simulink model "BlockDprob2f"  (R2016b)
settings: Solver=VariableStepAuto  StartTime=0.0  StopTime=230.0  RelTol=1e-3
values from neighbouring files (symbols this model uses):
  A = [-0.322, 0.052, 0.028, -1.12 , 0.002;       0     , 0    , 1    , -0.001,     0;       -10.6 , 0    , -2.87, 0.46  , -0.65;       6.87  , 0    , -0.04, -0.32 , -0.02;       0     , 0    , 0    , 0     ,   -10 ]    [run_task_2f.m]    (also in sys_matrices.m)
  a1 = 2.87    [run_task_2f.m]
  a2 = -0.65    [run_task_2f.m]
  B = [0 0 0 0 10]'    [run_task_2f.m]    (also in sys_matrices.m)
  C = [0 0 0 1 0;       0 0 1 0 0;       1 0 0 0 0;       0 1 0 0 0]    [run_task_2f.m]    (also in sys_matrices.m)
  d = 2    [run_task_2f.m]
  D = zeros(4,1)    [run_task_2f.m]
  g = 9.81    [run_task_2f.m]
  k_d_phi = f_kd(zp, wp)    [run_task_2f.m]
  k_i_chi = V_g/g * wx^2    [run_task_2f.m]
  k_i_phi = 0    [run_task_2f.m]
  k_p_chi = V_g/g * 2*zx*wx    [run_task_2f.m]
  k_p_phi = -5/3    (= -1.66666666667)    [run_task_2f.m]
  V_g = 637/3.6    (= 176.944444444)    [run_task_2f.m]
libraries: simulink_extras x7
settings Model: Creator=helene  LastModifiedBy=helene
settings ConfigComp: DVTestSuiteOptimization=CombinedObjectives (Nonlinear Extended)  DVDetectFloatOverflow=off

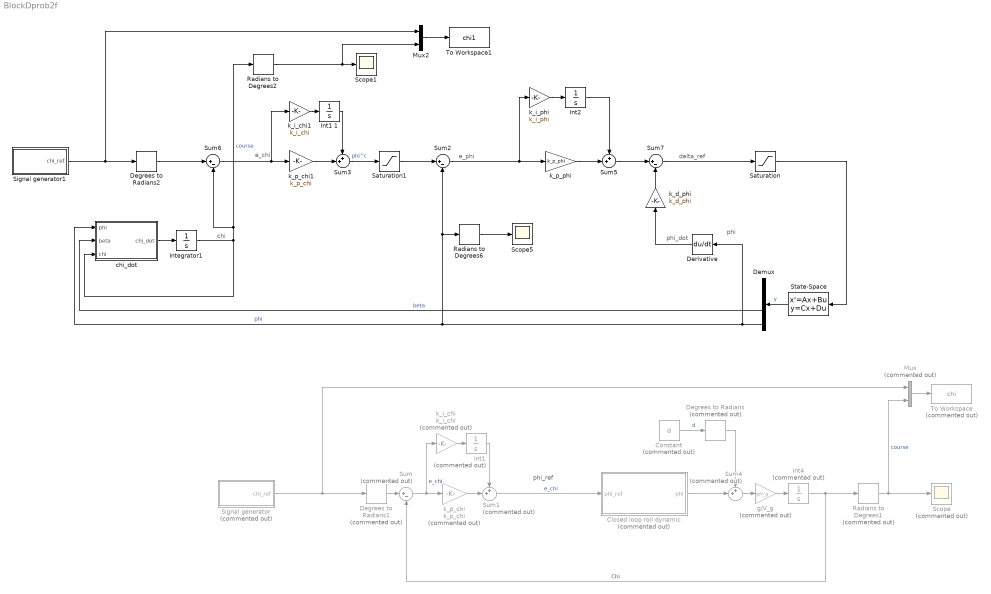
== system BlockDprob2f ==
  note: e_chi
  note: chi
  note: phi_dot
  note: e_phi
  note: phi
  note: delta_ref
  note: phi_ref
  Closed loop roll dynamic : Subsystem  Commented=on
  Constant : Constant  Commented=on  Value=d
  Degrees to Radians : simulink_extras/Transformations/Degrees to Radians  Commented=on
  Degrees to Radians1 : simulink_extras/Transformations/Degrees to Radians  Commented=on
  Degrees to Radians2 : simulink_extras/Transformations/Degrees to Radians
  Demux : Demux
  Derivative : Derivative
  "Int1 " : Integrator  Commented=on  UpperSaturationLimit=0.15  LowerSaturationLimit=-0.15
  Int1 1 : Integrator  LimitOutput=on  UpperSaturationLimit=0.15  LowerSaturationLimit=-0.15
  "Int2 " : Integrator
  Int4 : Integrator  Commented=on
  Integrator1 : Integrator
  Mux : Mux  Commented=on  Inputs=2
  Mux2 : Mux  Inputs=2
  Radians to Degrees1 : simulink_extras/Transformations/Radians to Degrees  Commented=on
  Radians to Degrees2 : simulink_extras/Transformations/Radians to Degrees
  Radians to Degrees6 : simulink_extras/Transformations/Radians to Degrees
  Saturation : Saturate  UpperLimit=25*deg2rad  LowerLimit=-25*deg2rad
  Saturation1 : Saturate  UpperLimit=4000*deg2rad  LowerLimit=-4000*deg2rad
  Scope : Scope  Commented=on
  Scope1 : Scope
  Scope5 : Scope
  Signal generator : Subsystem  Commented=on
  Signal generator1 : Subsystem
  State-Space : StateSpace  A=A  B=B  C=C  D=D  X0=0
  Sum : Sum  Commented=on  Inputs=|+-
  Sum1 : Sum  Commented=on  Inputs=++|
  Sum2 : Sum  Inputs=|+-
  Sum3 : Sum  Inputs=++|
  Sum4 : Sum  Commented=on  Inputs=++|
  Sum5 : Sum  Inputs=++|
  Sum6 : Sum  Inputs=|+-
  Sum7 : Sum  Inputs=|+-
  To Workspace : ToWorkspace  Commented=on  VariableName=chi  SaveFormat=Timeseries  SampleTime=-1
  To Workspace1 : ToWorkspace  VariableName=chi1  SaveFormat=Timeseries  SampleTime=-1
  chi_dot : MATLAB Function  TreatAsAtomicUnit=on
  g/V_g : Gain  Commented=on  Gain=g/V_g
  k_d_phi : Gain  Gain=k_d_phi
  k_i_chi : Gain  Commented=on  Gain=k_i_chi
  k_i_chi1 : Gain  Gain=k_i_chi
  k_i_phi : Gain  Gain=k_i_phi
  k_p_chi : Gain  Commented=on  Gain=k_p_chi
  k_p_chi1 : Gain  Gain=k_p_chi
  "k_p_phi " : Gain  Gain=k_p_phi
  wires:
  k_p_chi/1 -> Sum1/2
  Sum/1 -> k_p_chi/1, k_i_chi/1  "e_chi"
  k_i_chi/1 -> "Int1 "/1
  Sum4/1 -> g/V_g/1
  Int4/1 -> Radians to Degrees1/1, Sum/2  "Chi"
  Constant/1 -> Degrees to Radians/1  "d"
  g/V_g/1 -> Int4/1
  Radians to Degrees1/1 -> Mux/2, Scope/1  "course"
  Degrees to Radians/1 -> Sum4/1
  Degrees to Radians1/1 -> Sum/1
  "Int1 "/1 -> Sum1/1
  Mux/1 -> To Workspace/1
  Sum1/1 -> Closed loop roll dynamic/1(phi_ref)  "e_chi"
  Closed loop roll dynamic/1(phi) -> Sum4/2
  chi_dot/1(chi_dot) -> Integrator1/1
  k_i_phi/1 -> "Int2 "/1
  "Int2 "/1 -> Sum5/1
  "k_p_phi "/1 -> Sum5/2
  Sum2/1 -> k_i_phi/1, "k_p_phi "/1
  Sum3/1 -> Saturation1/1  "phi^c"
  Sum6/1 -> k_i_chi1/1, k_p_chi1/1
  k_p_chi1/1 -> Sum3/2
  k_i_chi1/1 -> Int1 1/1
  Int1 1/1 -> Sum3/1
  Derivative/1 -> k_d_phi/1
  k_d_phi/1 -> Sum7/2
  Signal generator/1(chi_ref) -> Mux/1, Degrees to Radians1/1
  Degrees to Radians2/1 -> Sum6/1
  Radians to Degrees2/1 -> Mux2/2, Scope1/1
  Radians to Degrees6/1 -> Scope5/1
  Demux/4 -> Derivative/1, Radians to Degrees6/1, Sum2/2, chi_dot/1(phi)  "phi"
  Saturation1/1 -> Sum2/1
  Mux2/1 -> To Workspace1/1
  Integrator1/1 -> chi_dot/3(chi), Radians to Degrees2/1, Sum6/2  "course"
  Sum5/1 -> Sum7/1
  Sum7/1 -> Saturation/1
  Saturation/1 -> State-Space/1
  State-Space/1 -> Demux/1  "y"
  Demux/3 -> chi_dot/2(beta)  "beta"
  Signal generator1/1(chi_ref) -> Mux2/1, Degrees to Radians2/1

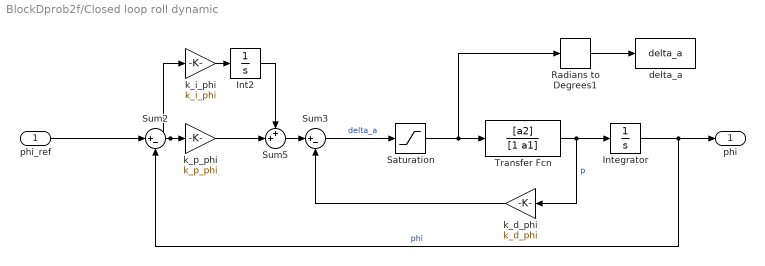
== system BlockDprob2f/Closed loop roll dynamic ==
  phi_ref : Inport
  "Int2 " : Integrator
  Integrator : Integrator
  Radians to Degrees1 : simulink_extras/Transformations/Radians to Degrees
  Saturation : Saturate  UpperLimit=25*deg2rad  LowerLimit=-25*deg2rad
  Sum2 : Sum  Inputs=|+-
  Sum3 : Sum  Inputs=|+-
  Sum5 : Sum  Inputs=++|
  Transfer Fcn : TransferFcn  Numerator=[a2]  Denominator=[1 a1]
  delta_a : ToWorkspace  VariableName=delta_a  SaveFormat=Timeseries  SampleTime=-1
  k_d_phi : Gain  Gain=k_d_phi
  k_i_phi : Gain  Gain=k_i_phi
  "k_p_phi " : Gain  Gain=k_p_phi
  phi : Outport
  wires:
  Sum2/1 -> k_i_phi/1, "k_p_phi "/1
  "k_p_phi "/1 -> Sum5/2
  k_i_phi/1 -> "Int2 "/1
  "Int2 "/1 -> Sum5/1
  Sum3/1 -> Saturation/1  "delta_a"
  k_d_phi/1 -> Sum3/2
  Integrator/1 -> phi/1, Sum2/2  "phi"
  Sum5/1 -> Sum3/1
  Transfer Fcn/1 -> Integrator/1, k_d_phi/1  "p"
  phi_ref/1 -> Sum2/1
  Saturation/1 -> Radians to Degrees1/1, Transfer Fcn/1
  Radians to Degrees1/1 -> delta_a/1

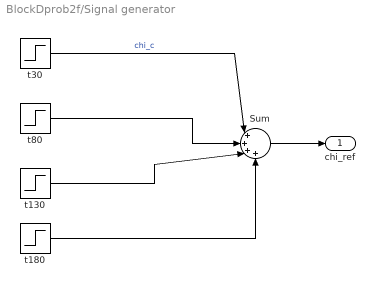
== system BlockDprob2f/Signal generator ==
  Sum : Sum  Inputs=|++++
  t130 : Step  Time=130  After=-15  SampleTime=0
  t180 : Step  Time=180  After=-10  SampleTime=0
  t30 : Step  Time=30  After=15  SampleTime=0
  "t80 " : Step  Time=80  After=10  SampleTime=0
  chi_ref : Outport
  wires:
  Sum/1 -> chi_ref/1
  t30/1 -> Sum/1  "chi_c"
  "t80 "/1 -> Sum/2
  t130/1 -> Sum/3
  t180/1 -> Sum/4

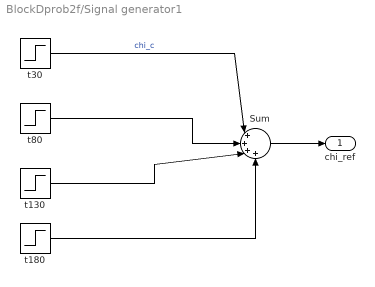
== system BlockDprob2f/Signal generator1 ==
  Sum : Sum  Inputs=|++++
  t130 : Step  Time=130  After=-15  SampleTime=0
  t180 : Step  Time=180  After=-10  SampleTime=0
  t30 : Step  Time=30  After=15  SampleTime=0
  "t80 " : Step  Time=80  After=10  SampleTime=0
  chi_ref : Outport
  wires:
  Sum/1 -> chi_ref/1
  t30/1 -> Sum/1  "chi_c"
  "t80 "/1 -> Sum/2
  t130/1 -> Sum/3
  t180/1 -> Sum/4

== matlab function BlockDprob2f/chi_dot ==
  data: phi input; beta input; chi input; chi_dot output
function chi_dot = fcn(phi,beta, chi)

d = 2 * pi/180;
g = 9.81; % [m/s^2] gravity
V_g = 637/3.6 ; % [m/s] Speed over ground (637 [km/h]) 

psi  = chi - beta;


chi_dot = g/V_g * tan(phi+d) *cos(chi - psi);
